simulink model "test"  (R2021b)
settings: Solver=VariableStepAuto  StartTime=0.0  StopTime=10.0  RelTol=1e-3
libraries: neural x1
settings Model: Creator=prostakk  LastModifiedBy=prostakk

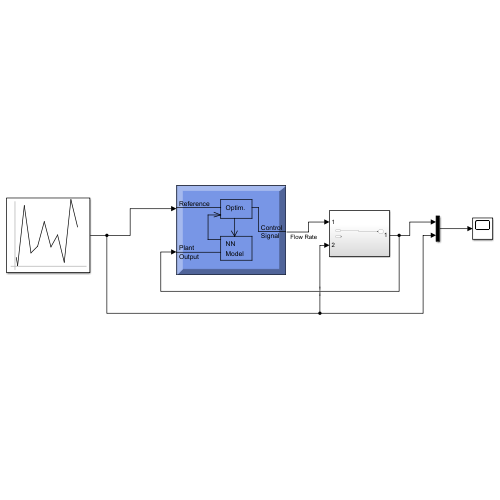
[thumbnail: Simulink's stored preview of the top-level diagram]
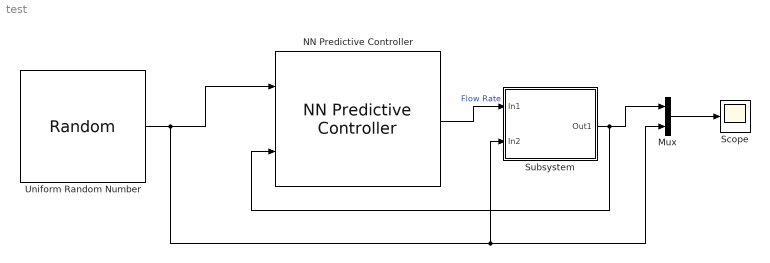
== system test ==
  Mux : Mux  Inputs=2
  NN Predictive Controller : neural/Control Systems/NN Predictive Controller  epochs=[]  minp=[]  maxp=[]  mint=[]  maxt=[]  Normalize=[]  IW=[]  LW1_2=[]  LW2_1=[]  B1=[]  B2=[]  max_i_int=[]  min_i_int=[]  limit_output=[]  max_output=[]  min_output=[]  Use_Previous_Weights=[]  N2=23  Nu=2  Ts=[]  rho=0.05  alpha=0.001  csrchfun=csrchbac  maxiter=2  S1=[]  Ni=[]  Nj=[]  sim_file=0  trainfun=trainlm  Use_validation=[]  Use_Testing=[]  max_i=[]  min_i=[]  sam_training=[]
      settings: SourceProductBaseCode=NN
  Scope : Scope
  Subsystem : Subsystem
  Uniform Random Number : UniformRandomNumber  SampleTime=0.1
  wires:
  Uniform Random Number/1 -> Subsystem/2(In2), Mux/2, NN Predictive Controller/1
  Mux/1 -> Scope/1
  Subsystem/1(Out1) -> NN Predictive Controller/2, Mux/1
  NN Predictive Controller/1 -> Subsystem/1(In1)  "Flow Rate"

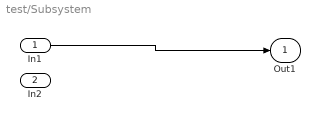
== system test/Subsystem ==
  In1 : Inport
  In2 : Inport  Port=2
  Out1 : Outport
  wires:
  In1/1 -> Out1/1
